simulink model "controller_simulation"  (R2022b)
settings: Solver=VariableStepAuto  StartTime=0.0  StopTime=10.0  FixedStep=0.005  RelTol=1e-3
values from neighbouring files (symbols this model uses):
  A = [0,  0,                             1,                           0 ... (first row only)    [main.m]    (also in taak.m = [0, 0, 1, 0; 0, 0, 0, 1; 0, K_stiff/J_h, -((K_g)^2*K_m*K_b)/)
  B = [ 0 ... (first row only)    [main.m]    (also in taak.m = [0; 0; (K_m*K_g)/(R_m*J_h);-(K_m*K_g)/(R_m*J_h)])
  C = [1 0 0 0 ... (first row only)    [main.m]
  D = zeros(2,1)    [main.m]
  Ts = 1/200    (= 0.005)    [main.m]
  w_c = 2*2*pi    (= 12.5663706144)    [main.m]
undefined symbols (not defined in the file or in its folder): K
settings Model: Creator=Sofie  LastModifiedBy=Sofie

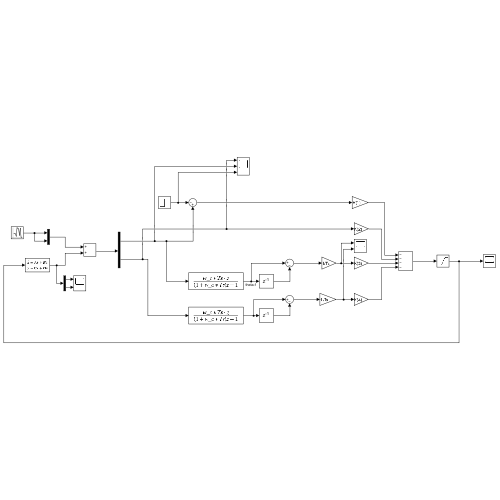
[thumbnail: Simulink's stored preview of the top-level diagram]
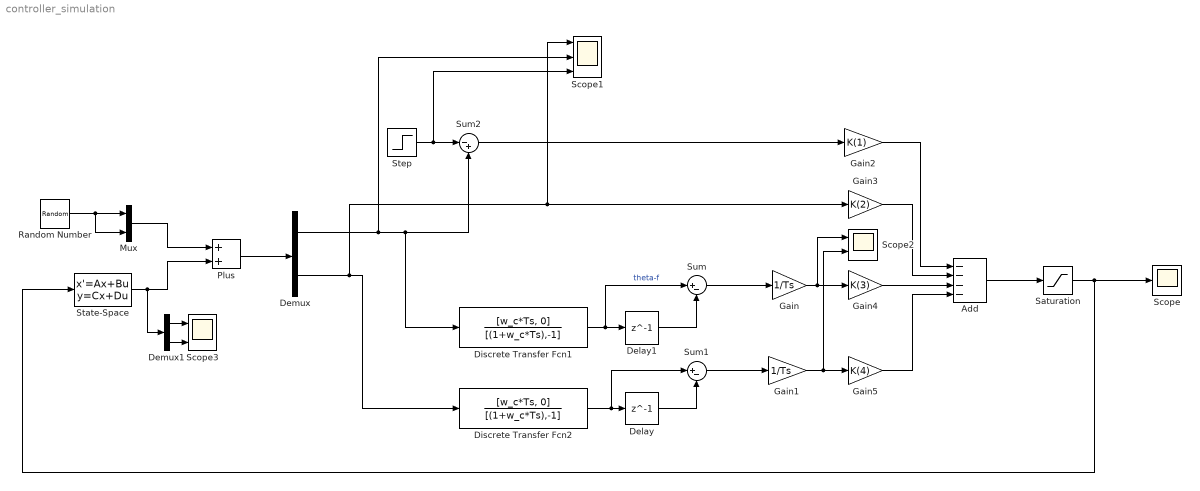
== system controller_simulation ==
  Add : Sum  Inputs=----
  Delay : Delay  DelayLength=1
  Delay1 : Delay  DelayLength=1
  Demux : Demux  Outputs=2
  Demux1 : Demux  Outputs=2
  Discrete Transfer Fcn1 : DiscreteTransferFcn  Numerator=[w_c*Ts, 0]  Denominator=[(1+w_c*Ts),-1]  SampleTime=Ts
  Discrete Transfer Fcn2 : DiscreteTransferFcn  Numerator=[w_c*Ts, 0]  Denominator=[(1+w_c*Ts),-1]  SampleTime=Ts
  Gain : Gain  Gain=1/Ts
  Gain1 : Gain  Gain=1/Ts
  Gain2 : Gain  Gain=K(1)
  Gain3 : Gain  Gain=K(2)
  Gain4 : Gain  Gain=K(3)
  Gain5 : Gain  Gain=K(4)
  Mux : Mux  Inputs=2
  Plus : Sum
  Random Number : RandomNumber  Variance=0.005  SampleTime=1/200
  Saturation : Saturate  UpperLimit=5  LowerLimit=-5
  Scope : Scope
  Scope1 : Scope  NumInputPorts=3
  Scope2 : Scope  NumInputPorts=2
  Scope3 : Scope  NumInputPorts=2
  State-Space : StateSpace  A=A  B=B  C=C  D=D  InitialCondition=0
  Step : Step  Time=5  After=pi/2  SampleTime=0
  Sum : Sum  Inputs=|+-
  Sum1 : Sum  Inputs=|+-
  Sum2 : Sum  Inputs=|-+
  wires:
  Demux/1 -> Scope1/2, Sum2/2, Discrete Transfer Fcn1/1
  Demux/2 -> Scope1/1, Gain3/1, Discrete Transfer Fcn2/1
  Random Number/1 -> Mux/2, Mux/1
  Mux/1 -> Plus/1
  State-Space/1 -> Demux1/1, Plus/2
  Plus/1 -> Demux/1
  Discrete Transfer Fcn1/1 -> Sum/1, Delay1/1  "theta-f"
  Delay1/1 -> Sum/2
  Delay/1 -> Sum1/2
  Discrete Transfer Fcn2/1 -> Sum1/1, Delay/1
  Sum/1 -> Gain/1
  Sum1/1 -> Gain1/1
  Sum2/1 -> Gain2/1
  Step/1 -> Scope1/3, Sum2/1
  Gain1/1 -> Scope2/2, Gain5/1
  Gain2/1 -> Add/1
  Gain3/1 -> Add/2
  Gain4/1 -> Add/3
  Gain5/1 -> Add/4
  Add/1 -> Saturation/1
  Saturation/1 -> Scope/1, State-Space/1
  Gain/1 -> Scope2/1, Gain4/1
  Demux1/2 -> Scope3/2
  Demux1/1 -> Scope3/1
